simulink model "Quad_Nonlinear_Roll_LQIDG_Model"  (R2020a)
settings: Solver=ode4  StartTime=0.0  StopTime=20  FixedStep=0.02  RelTol=1e-3
InitFcn:
  | OpenLoop_LQDG_riccati_solver_roll;
values from neighbouring files (symbols this model uses):
  LQIDG_openloop_gain = (R1_inv * B' * p1)    [OpenLoop_LQDG_riccati_solver_roll.m]
undefined symbols (not defined in the file or in its folder): A6, DiscIntNeverNeededParam, g, h_cg, J_xx, m1, m_tot, miu_k, r_x
libraries: simulink x1, eeGeneralControl x1
settings Model: Creator=Ali  LastModifiedBy=Ali

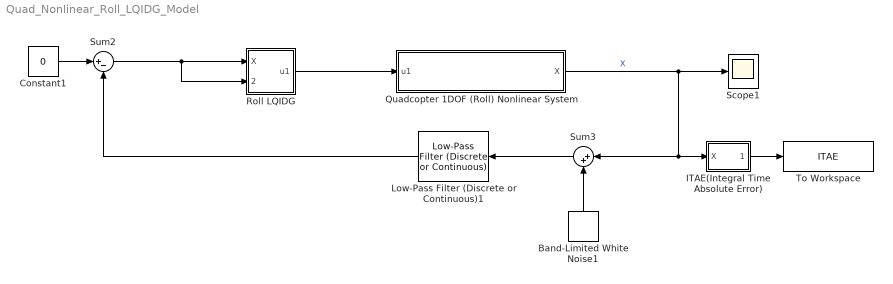
== system Quad_Nonlinear_Roll_LQIDG_Model ==
  Band-Limited White Noise1 : simulink/Sources/Band-Limited White Noise  Cov=[0.0005]  Ts=0.02  seed=[23341]
  Constant1 : Constant  Value=0
  ITAE(Integral Time Absolute Error) : Subsystem
  Low-Pass Filter (Discrete or Continuous)1 : eeGeneralControl/Low-Pass Filter (Discrete or Continuous)  K=1  T=0.01  B=inf  A=-inf  init_option=Inherited from block input  x0=0  Ts=-1
  Quadcopter 1DOF (Roll) Nonlinear System : Subsystem  TreatAsAtomicUnit=on
  Roll LQIDG : Subsystem
  Scope1 : Scope
  Sum2 : Sum  Inputs=|+-
  Sum3 : Sum  Inputs=|++
  To Workspace : ToWorkspace  VariableName=ITAE  SaveFormat=Timeseries  SampleTime=-1
  wires:
  Roll LQIDG/1(u1) -> Quadcopter 1DOF (Roll) Nonlinear System/1(u1)
  Band-Limited White Noise1/1 -> Sum3/2
  ITAE(Integral Time Absolute Error)/1(ITAE) -> To Workspace/1
  Sum3/1 -> Low-Pass Filter (Discrete or Continuous)1/1
  Sum2/1 -> Roll LQIDG/2(Error), Roll LQIDG/1(X)
  Low-Pass Filter (Discrete or Continuous)1/1 -> Sum2/2
  Quadcopter 1DOF (Roll) Nonlinear System/1(X) -> Sum3/1, ITAE(Integral Time Absolute Error)/1(X), Scope1/1  "X"
  Constant1/1 -> Sum2/1

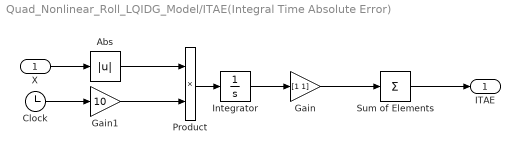
== system Quad_Nonlinear_Roll_LQIDG_Model/ITAE(Integral Time Absolute Error) ==
  X : Inport
  Abs : Abs
  Clock : Clock
  Gain : Gain  Gain=[1 1]
  Gain1 : Gain  Gain=10
  Integrator : Integrator
  Product : Product
  Sum of Elements : Sum  Inputs=+
  ITAE : Outport
  wires:
  Product/1 -> Integrator/1
  Integrator/1 -> Gain/1
  Clock/1 -> Gain1/1
  Sum of Elements/1 -> ITAE/1
  Abs/1 -> Product/1
  X/1 -> Abs/1
  Gain/1 -> Sum of Elements/1
  Gain1/1 -> Product/2

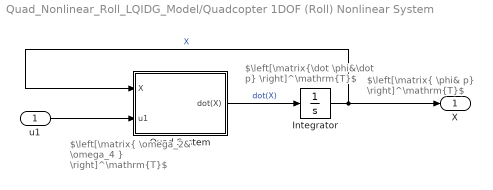
== system Quad_Nonlinear_Roll_LQIDG_Model/Quadcopter 1DOF (Roll) Nonlinear System ==
  note: $\left[\matrix{ \phi& p} \right]^\mathrm{T}$
  note: $\left[\matrix{ \omega_2& \omega_4 } \right]^\mathrm{T}$
  note: $\left[\matrix{\dot \phi&\dot p} \right]^\mathrm{T}$
  u1 : Inport
  Integrator : Integrator  InitialCondition=[5*pi/180, -5*pi/180]
  Quad System : Subsystem
  X : Outport
  wires:
  Integrator/1 -> Quad System/1(X), X/1  "X"
  Quad System/1(dot(X)) -> Integrator/1  "dot(X)"
  u1/1 -> Quad System/2(u1)

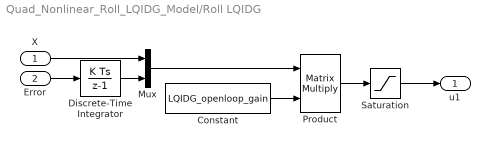
== system Quad_Nonlinear_Roll_LQIDG_Model/Roll LQIDG ==
  X : Inport
  Error : Inport  Port=2
  Constant : Constant  Value=LQIDG_openloop_gain
  Discrete-Time Integrator : DiscreteIntegrator  SampleTime=-1  LimitOutput=on  UpperSaturationLimit=1.5  LowerSaturationLimit=-1.5  ICPrevOutput=DiscIntNeverNeededParam  ICPrevScaledInput=DiscIntNeverNeededParam
  Mux : Mux  Inputs=2
  Product : Product  Multiplication=Matrix(*)
  Saturation : Saturate  UpperLimit=12  LowerLimit=-12
  u1 : Outport
  wires:
  Product/1 -> Saturation/1
  Constant/1 -> Product/2
  X/1 -> Mux/1
  Error/1 -> Discrete-Time Integrator/1
  Mux/1 -> Product/1
  Discrete-Time Integrator/1 -> Mux/2
  Saturation/1 -> u1/1

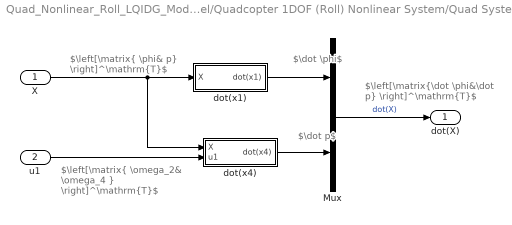
== system Quad_Nonlinear_Roll_LQIDG_Model/Quadcopter 1DOF (Roll) Nonlinear System/Quad System ==
  note: $\dot \phi$
  note: $\left[\matrix{ \omega_2& \omega_4 } \right]^\mathrm{T}$
  note: $\left[\matrix{ \phi& p} \right]^\mathrm{T}$
  note: $\left[\matrix{\dot \phi&\dot p} \right]^\mathrm{T}$
  note: $\dot p$
  X : Inport
  u1 : Inport  Port=2
  Mux : Mux  Inputs=2
  dot(x1) : Subsystem
  dot(x4) : Subsystem
  dot(X) : Outport
  wires:
  Mux/1 -> dot(X)/1  "dot(X)"
  X/1 -> dot(x4)/1(X), dot(x1)/1(X)
  u1/1 -> dot(x4)/2(u1)
  dot(x1)/1(dot(x1)) -> Mux/1
  dot(x4)/1(dot(x4)) -> Mux/2

== system Quad_Nonlinear_Roll_LQIDG_Model/Quadcopter 1DOF (Roll) Nonlinear System/Quad System/dot(x1) ==
  X : Inport
  Subsystem1 : Subsystem
  dot(x1) : Outport
  wires:
  X/1 -> Subsystem1/1(X)  "X"
  Subsystem1/1(x4) -> dot(x1)/1

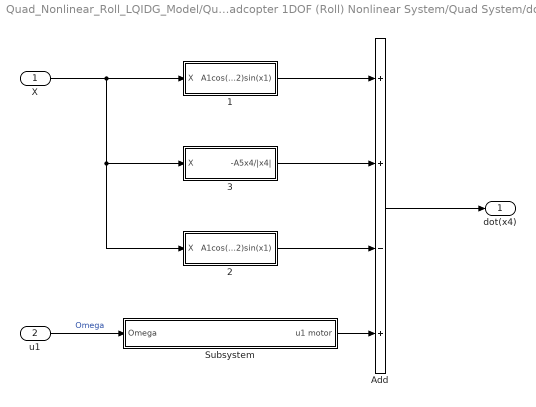
== system Quad_Nonlinear_Roll_LQIDG_Model/Quadcopter 1DOF (Roll) Nonlinear System/Quad System/dot(x4) ==
  X : Inport
  u1 : Inport  Port=2
  1 : Subsystem
  2 : Subsystem
  3 : Subsystem
  Add : Sum  Inputs=++-+
  Subsystem : Subsystem
  dot(x4) : Outport
  wires:
  u1/1 -> Subsystem/1(Omega)  "Omega"
  Add/1 -> dot(x4)/1
  1/1(A1cos(x2)sin(x1)) -> Add/1
  3/1("-A5x4/|x4| ") -> Add/2
  X/1 -> 2/1(X), 3/1(X), 1/1(X)
  Subsystem/1(u1 motor) -> Add/4
  2/1(A1cos(x2)sin(x1)) -> Add/3

== system Quad_Nonlinear_Roll_LQIDG_Model/Quadcopter 1DOF (Roll) Nonlinear System/Quad System/dot(x1)/Subsystem1 ==
  X : Inport
  Selector : Selector  InputPortWidth=2  IndexOptions=Index vector (dialog)  Indices=[2]  OutputSizes=1
  x4 : Outport
  wires:
  Selector/1 -> x4/1
  X/1 -> Selector/1

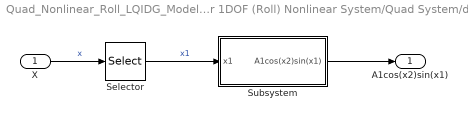
== system Quad_Nonlinear_Roll_LQIDG_Model/Quadcopter 1DOF (Roll) Nonlinear System/Quad System/dot(x4)/1 ==
  X : Inport
  Selector : Selector  InputPortWidth=2  IndexOptions=Index vector (dialog)  Indices=[1]  OutputSizes=1
  Subsystem : Subsystem
  A1cos(x2)sin(x1) : Outport
  wires:
  Selector/1 -> Subsystem/1(x1)  "x1"
  Subsystem/1(A1cos(x2)sin(x1)) -> A1cos(x2)sin(x1)/1
  X/1 -> Selector/1  "x"

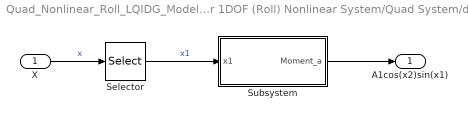
== system Quad_Nonlinear_Roll_LQIDG_Model/Quadcopter 1DOF (Roll) Nonlinear System/Quad System/dot(x4)/2 ==
  X : Inport
  Selector : Selector  InputPortWidth=2  IndexOptions=Index vector (dialog)  Indices=[1]  OutputSizes=1
  Subsystem : Subsystem
  A1cos(x2)sin(x1) : Outport
  wires:
  Selector/1 -> Subsystem/1(x1)  "x1"
  Subsystem/1(Moment_a) -> A1cos(x2)sin(x1)/1
  X/1 -> Selector/1  "x"

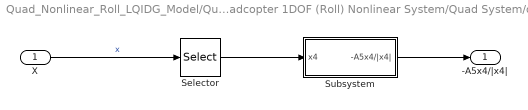
== system Quad_Nonlinear_Roll_LQIDG_Model/Quadcopter 1DOF (Roll) Nonlinear System/Quad System/dot(x4)/3 ==
  X : Inport
  Selector : Selector  InputPortWidth=2  IndexOptions=Index vector (dialog)  Indices=[2]  OutputSizes=1
  Subsystem : Subsystem
  "-A5x4/|x4| " : Outport
  wires:
  Subsystem/1("-A5x4/|x4| ") -> "-A5x4/|x4| "/1
  X/1 -> Selector/1  "x"
  Selector/1 -> Subsystem/1(x4)

== system Quad_Nonlinear_Roll_LQIDG_Model/Quadcopter 1DOF (Roll) Nonlinear System/Quad System/dot(x4)/Subsystem ==
  Omega : Inport
  Delay : Delay  DelayLength=1
  Transfer Fcn : TransferFcn  Denominator=[0.15 1]
  u1 motor : Outport
  wires:
  Omega/1 -> Delay/1
  Delay/1 -> Transfer Fcn/1
  Transfer Fcn/1 -> u1 motor/1

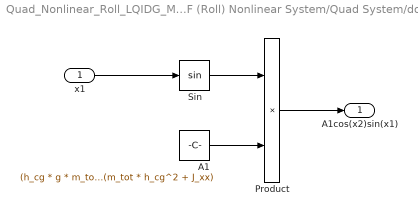
== system Quad_Nonlinear_Roll_LQIDG_Model/Quadcopter 1DOF (Roll) Nonlinear System/Quad System/dot(x4)/1/Subsystem ==
  x1 : Inport
  A1 : Constant  Value=(h_cg * g * m_tot) / (m_tot * h_cg^2 + J_xx)
  Product : Product
  Sin : Trigonometry
  A1cos(x2)sin(x1) : Outport
  wires:
  Sin/1 -> Product/1
  Product/1 -> A1cos(x2)sin(x1)/1
  x1/1 -> Sin/1
  A1/1 -> Product/2

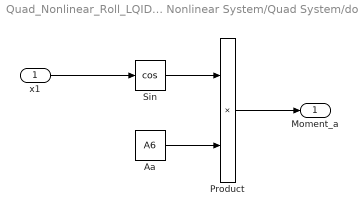
== system Quad_Nonlinear_Roll_LQIDG_Model/Quadcopter 1DOF (Roll) Nonlinear System/Quad System/dot(x4)/2/Subsystem ==
  x1 : Inport
  Aa : Constant  Value=A6
  Product : Product
  Sin : Trigonometry  Operator=cos
  Moment_a : Outport
  wires:
  Sin/1 -> Product/1
  Product/1 -> Moment_a/1
  x1/1 -> Sin/1
  Aa/1 -> Product/2

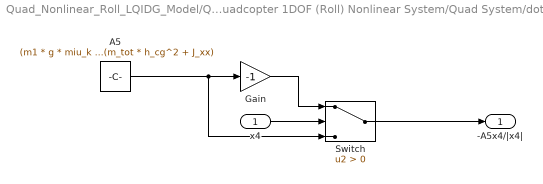
== system Quad_Nonlinear_Roll_LQIDG_Model/Quadcopter 1DOF (Roll) Nonlinear System/Quad System/dot(x4)/3/Subsystem ==
  x4 : Inport
  A5 : Constant  Value=(m1 * g * miu_k * r_x) / (m_tot * h_cg^2 + J_xx)
  Gain : Gain  Gain=-1
  Switch : Switch  Criteria=u2 > Threshold
  "-A5x4/|x4| " : Outport
  wires:
  Switch/1 -> "-A5x4/|x4| "/1
  A5/1 -> Switch/3, Gain/1
  x4/1 -> Switch/2
  Gain/1 -> Switch/1
